simulink model "Lv_topo4"  (R2024a)
settings: Solver=ode4  StartTime=0.0  StopTime=1  FixedStep=5e-05  RelTol=1e-3
libraries: spsSeriesRLCBranchLib x38, spsThreePhaseSeriesRLCBranchLib x18, spsCurrentMeasurementLib x16, spsPowerLib x16, spsSeriesRLCLoadLib x16, spsVoltageMeasurementLib x16, spsThreePhaseVIMeasurementLib x2, spsGroundLib x2, spsPower3phInstantaneousLib x2, spsThreePhaseTransformerTwoWindingsLib x2, spsThreePhaseSourceLib x1, sps_lib x1
(part 1 of 2)
settings Model: SimulationMode=accelerator  Creator=zyx53  LastModifiedBy=zyx53
settings DataIOCC: SaveFinalState=on  SaveOperatingPoint=on  SaveState=on  ReturnWorkspaceOutputs=off

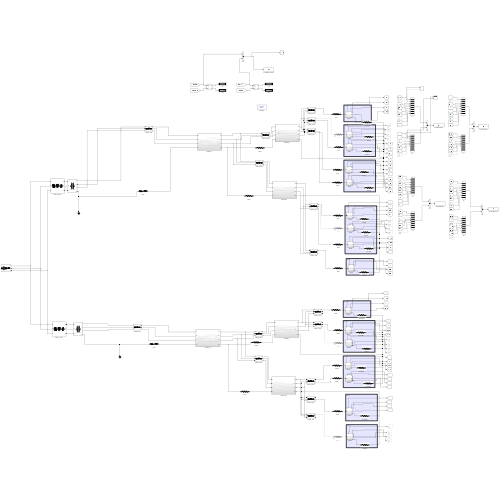
[thumbnail: Simulink's stored preview of the top-level diagram]
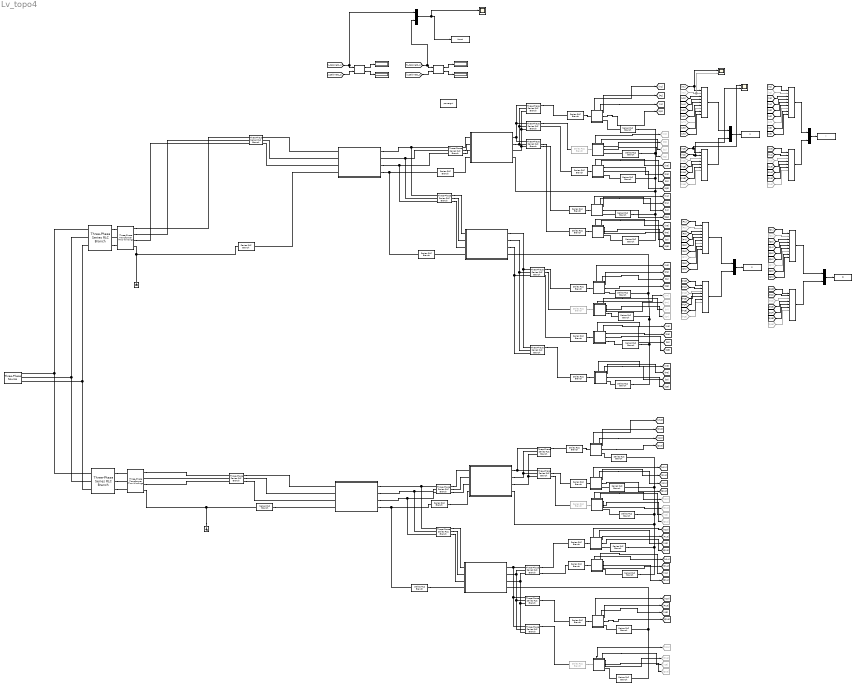
== system Lv_topo4 ==
  note: 表箱1
  note: 表箱2
  note: 表箱3
  note: 表箱4
  note: 表箱5
  note: 表箱1
  note: 表箱2
  note: 表箱3
  note: 表箱4
  note: 表箱5
  10+10m{1..2,21..22} (4 alike) : spsSeriesRLCBranchLib/Series RLC Branch  LConnTagsString=__new0  RConnTagsString=__new0  BranchType=R  Resistance=20*3.08e-3  Inductance=0  SetiL0=off  InitialCurrent=0  Capacitance=1e-6  Setx0=off  InitialVoltage=0  Measurements=None
  10+15m21 : spsSeriesRLCBranchLib/Series RLC Branch  LConnTagsString=__new0  RConnTagsString=__new0  BranchType=R  Resistance=25*3.08e-3  Inductance=0  SetiL0=off  InitialCurrent=0  Capacitance=1e-6  Setx0=off  InitialVoltage=0  Measurements=None
  10+15m24 : spsSeriesRLCBranchLib/Series RLC Branch  LConnTagsString=__new0  RConnTagsString=__new0  BranchType=R  Resistance=25*3.08e-3  Inductance=0  SetiL0=off  InitialCurrent=0  Capacitance=1e-6  Setx0=off  InitialVoltage=0  Measurements=None
  10+15m3 : spsSeriesRLCBranchLib/Series RLC Branch  LConnTagsString=__new0  RConnTagsString=__new0  BranchType=R  Resistance=25*3.08e-3  Inductance=0  SetiL0=off  InitialCurrent=0  Capacitance=1e-6  Setx0=off  InitialVoltage=0  Measurements=None
  10+5m{1..3,5,7,23} (6 alike) : spsSeriesRLCBranchLib/Series RLC Branch  LConnTagsString=__new0  RConnTagsString=__new0  BranchType=R  Resistance=15*3.08e-3  Inductance=0  SetiL0=off  InitialCurrent=0  Capacitance=1e-6  Setx0=off  InitialVoltage=0  Measurements=None
  10+7m2 : spsSeriesRLCBranchLib/Series RLC Branch  LConnTagsString=__new0  RConnTagsString=__new0  BranchType=R  Resistance=17*3.08e-3  Inductance=0  SetiL0=off  InitialCurrent=0  Capacitance=1e-6  Setx0=off  InitialVoltage=0  Measurements=None
  10m : spsSeriesRLCBranchLib/Series RLC Branch  LConnTagsString=__new0  RConnTagsString=__new0  BranchType=R  Resistance=10*3.08e-3  Inductance=0  SetiL0=off  InitialCurrent=0  Capacitance=1e-6  Setx0=off  InitialVoltage=0  Measurements=None
  10m1 : spsSeriesRLCBranchLib/Series RLC Branch  LConnTagsString=__new0  RConnTagsString=__new0  BranchType=R  Resistance=10*3.08e-3  Inductance=0  SetiL0=off  InitialCurrent=0  Capacitance=1e-6  Setx0=off  InitialVoltage=0  Measurements=None
  10m2 : spsSeriesRLCBranchLib/Series RLC Branch  LConnTagsString=__new0  RConnTagsString=__new0  BranchType=R  Resistance=10*3.08e-3  Inductance=0  SetiL0=off  InitialCurrent=0  Capacitance=1e-6  Setx0=off  InitialVoltage=0  Measurements=None
  10m21 : spsSeriesRLCBranchLib/Series RLC Branch  LConnTagsString=__new0  RConnTagsString=__new0  BranchType=R  Resistance=10*3.08e-3  Inductance=1.4e-5  SetiL0=off  InitialCurrent=0  Capacitance=1e-6  Setx0=off  InitialVoltage=0  Measurements=None
  10m22 : spsSeriesRLCBranchLib/Series RLC Branch  LConnTagsString=__new0  RConnTagsString=__new0  BranchType=R  Resistance=10*3.08e-3  Inductance=1.04e-5  SetiL0=off  InitialCurrent=0  Capacitance=1e-6  Setx0=off  InitialVoltage=0  Measurements=None
  10m24 : spsSeriesRLCBranchLib/Series RLC Branch  LConnTagsString=__new0  RConnTagsString=__new0  BranchType=R  Resistance=10*3.08e-3  Inductance=7.6e-6  SetiL0=off  InitialCurrent=0  Capacitance=1e-6  Setx0=off  InitialVoltage=0  Measurements=None
  10m26 : spsSeriesRLCBranchLib/Series RLC Branch  Commented=on  LConnTagsString=__new0  RConnTagsString=__new0  BranchType=R  Resistance=10*3.08e-3  Inductance=9.6e-6  SetiL0=off  InitialCurrent=0  Capacitance=1e-6  Setx0=off  InitialVoltage=0  Measurements=None
  10m27 : spsSeriesRLCBranchLib/Series RLC Branch  LConnTagsString=__new0  RConnTagsString=__new0  BranchType=R  Resistance=10*3.08e-3  Inductance=1.2e-5  SetiL0=off  InitialCurrent=0  Capacitance=1e-6  Setx0=off  InitialVoltage=0  Measurements=None
  10m5 : spsSeriesRLCBranchLib/Series RLC Branch  LConnTagsString=__new0  RConnTagsString=__new0  BranchType=R  Resistance=10*3.08e-3  Inductance=8.8e-6  SetiL0=off  InitialCurrent=0  Capacitance=1e-6  Setx0=off  InitialVoltage=0  Measurements=None
  10m7 : spsSeriesRLCBranchLib/Series RLC Branch  LConnTagsString=__new0  RConnTagsString=__new0  BranchType=R  Resistance=10*3.08e-3  Inductance=6e-6  SetiL0=off  InitialCurrent=0  Capacitance=1e-6  Setx0=off  InitialVoltage=0  Measurements=None
  20m1 : spsSeriesRLCBranchLib/Series RLC Branch  LConnTagsString=__new0  RConnTagsString=__new0  BranchType=R  Resistance=10*3.08e-3  Inductance=0  SetiL0=off  InitialCurrent=0  Capacitance=1e-6  Setx0=off  InitialVoltage=0  Measurements=None
  20m3 : spsSeriesRLCBranchLib/Series RLC Branch  LConnTagsString=__new0  RConnTagsString=__new0  BranchType=R  Resistance=20*3.08e-3  Inductance=0  SetiL0=off  InitialCurrent=0  Capacitance=1e-6  Setx0=off  InitialVoltage=0  Measurements=None
  25m21 : spsSeriesRLCBranchLib/Series RLC Branch  LConnTagsString=__new0  RConnTagsString=__new0  BranchType=R  Resistance=25*3.08e-3  Inductance=0  SetiL0=off  InitialCurrent=0  Capacitance=1e-6  Setx0=off  InitialVoltage=0  Measurements=None
  30m2 : spsSeriesRLCBranchLib/Series RLC Branch  LConnTagsString=__new0  RConnTagsString=__new0  BranchType=R  Resistance=30*3.08e-3  Inductance=0  SetiL0=off  InitialCurrent=0  Capacitance=1e-6  Setx0=off  InitialVoltage=0  Measurements=None
  3m2 : spsSeriesRLCBranchLib/Series RLC Branch  LConnTagsString=__new0  RConnTagsString=__new0  BranchType=RL  Resistance=0.00549  Inductance=1.2e-5  SetiL0=off  InitialCurrent=0  Capacitance=1e-6  Setx0=off  InitialVoltage=0  Measurements=None
  3m5 : spsSeriesRLCBranchLib/Series RLC Branch  LConnTagsString=__new0  RConnTagsString=__new0  BranchType=RL  Resistance=0.00549  Inductance=1.2e-5  SetiL0=off  InitialCurrent=0  Capacitance=1e-6  Setx0=off  InitialVoltage=0  Measurements=None
  5+15m25 : spsSeriesRLCBranchLib/Series RLC Branch  LConnTagsString=__new0  RConnTagsString=__new0  BranchType=R  Resistance=20*3.08e-3  Inductance=0  SetiL0=off  InitialCurrent=0  Capacitance=1e-6  Setx0=off  InitialVoltage=0  Measurements=None
  5+5m1 : spsSeriesRLCBranchLib/Series RLC Branch  LConnTagsString=__new0  RConnTagsString=__new0  BranchType=R  Resistance=10*3.08e-3  Inductance=0  SetiL0=off  InitialCurrent=0  Capacitance=1e-6  Setx0=off  InitialVoltage=0  Measurements=None
  5m : spsSeriesRLCBranchLib/Series RLC Branch  Commented=on  LConnTagsString=__new0  RConnTagsString=__new0  BranchType=R  Resistance=5*3.08e-3  Inductance=0  SetiL0=off  InitialCurrent=0  Capacitance=1e-6  Setx0=off  InitialVoltage=0  Measurements=None
  5m2 : spsSeriesRLCBranchLib/Series RLC Branch  LConnTagsString=__new0  RConnTagsString=__new0  BranchType=R  Resistance=5*3.08e-3  Inductance=0  SetiL0=off  InitialCurrent=0  Capacitance=1e-6  Setx0=off  InitialVoltage=0  Measurements=None
  5m23 : spsSeriesRLCBranchLib/Series RLC Branch  Commented=on  LConnTagsString=__new0  RConnTagsString=__new0  BranchType=R  Resistance=5*3.08e-3  Inductance=9.2e-6  SetiL0=off  InitialCurrent=0  Capacitance=1e-6  Setx0=off  InitialVoltage=0  Measurements=None
  5m25 : spsSeriesRLCBranchLib/Series RLC Branch  LConnTagsString=__new0  RConnTagsString=__new0  BranchType=R  Resistance=5*3.08e-3  Inductance=4.4e-6  SetiL0=off  InitialCurrent=0  Capacitance=1e-6  Setx0=off  InitialVoltage=0  Measurements=None
  5m3 : spsSeriesRLCBranchLib/Series RLC Branch  LConnTagsString=__new0  RConnTagsString=__new0  BranchType=R  Resistance=5*3.08e-3  Inductance=0  SetiL0=off  InitialCurrent=0  Capacitance=1e-6  Setx0=off  InitialVoltage=0  Measurements=None
  7m1 : spsSeriesRLCBranchLib/Series RLC Branch  Commented=on  LConnTagsString=__new0  RConnTagsString=__new0  BranchType=R  Resistance=7*3.08e-3  Inductance=1.2e-5  SetiL0=off  InitialCurrent=0  Capacitance=1e-6  Setx0=off  InitialVoltage=0  Measurements=None
  Cabinet1_1 : Subsystem
  Cabinet1_2 : Subsystem
  Cabinet2_1 : Subsystem
  Cabinet2_2 : Subsystem
  Cabinet2_3 : Subsystem
  Cabinet2_4 : Subsystem
  Cable1_10m1 : spsThreePhaseSeriesRLCBranchLib/Three-Phase Series RLC Branch  LConnTagsString=A|B|C  RConnTagsString=A|B|C  BranchType=RLC  Resistance=10*1.1e-7  Inductance=10*3.9e-8  Capacitance=0  Measurements=None
  Cable1_10m3 : spsThreePhaseSeriesRLCBranchLib/Three-Phase Series RLC Branch  LConnTagsString=A|B|C  RConnTagsString=A|B|C  BranchType=RLC  Resistance=10*1.1e-7  Inductance=10*3.9e-8  Capacitance=0  Measurements=None
  Cable1_10m5 : spsThreePhaseSeriesRLCBranchLib/Three-Phase Series RLC Branch  LConnTagsString=A|B|C  RConnTagsString=A|B|C  BranchType=RLC  Resistance=10*1.1e-7  Inductance=10*3.9e-8  Capacitance=0  Measurements=None
  Cable1_10m6 : spsThreePhaseSeriesRLCBranchLib/Three-Phase Series RLC Branch  LConnTagsString=A|B|C  RConnTagsString=A|B|C  BranchType=RLC  Resistance=15*1.1e-7  Inductance=15*3.9e-8  Capacitance=0  Measurements=None
  Cable1_15m1 : spsThreePhaseSeriesRLCBranchLib/Three-Phase Series RLC Branch  LConnTagsString=A|B|C  RConnTagsString=A|B|C  BranchType=RLC  Resistance=15*1.1e-7  Inductance=15*3.9e-8  Capacitance=0  Measurements=None
  Cable1_15m2 : spsThreePhaseSeriesRLCBranchLib/Three-Phase Series RLC Branch  LConnTagsString=A|B|C  RConnTagsString=A|B|C  BranchType=RLC  Resistance=15*1.1e-7  Inductance=15*3.9e-8  Capacitance=0  Measurements=None
  Cable1_15m3 : spsThreePhaseSeriesRLCBranchLib/Three-Phase Series RLC Branch  LConnTagsString=A|B|C  RConnTagsString=A|B|C  BranchType=RLC  Resistance=1.31e-3  Inductance=1.07e-3  Capacitance=0  Measurements=None
  Cable1_15m4 : spsThreePhaseSeriesRLCBranchLib/Three-Phase Series RLC Branch  LConnTagsString=A|B|C  RConnTagsString=A|B|C  BranchType=RLC  Resistance=1.31e-3  Inductance=1.07e-3  Capacitance=0  Measurements=None
  Cable1_15m5 : spsThreePhaseSeriesRLCBranchLib/Three-Phase Series RLC Branch  LConnTagsString=A|B|C  RConnTagsString=A|B|C  BranchType=RLC  Resistance=15*1.1e-7  Inductance=15*3.9e-8  Capacitance=0  Measurements=None
  Cable1_25m1 : spsThreePhaseSeriesRLCBranchLib/Three-Phase Series RLC Branch  LConnTagsString=A|B|C  RConnTagsString=A|B|C  BranchType=RLC  Resistance=25*1.1e-7  Inductance=25*3.9e-8  Capacitance=0  Measurements=None
  Cable1_30m2 : spsThreePhaseSeriesRLCBranchLib/Three-Phase Series RLC Branch  LConnTagsString=A|B|C  RConnTagsString=A|B|C  BranchType=RLC  Resistance=30*1.1e-7  Inductance=30*3.9e-8  Capacitance=0  Measurements=None
  Cable1_3m2 : spsThreePhaseSeriesRLCBranchLib/Three-Phase Series RLC Branch  LConnTagsString=A|B|C  RConnTagsString=A|B|C  BranchType=RLC  Resistance=0.000804  Inductance=0  Capacitance=0  Measurements=None
  Cable1_5m1 : spsThreePhaseSeriesRLCBranchLib/Three-Phase Series RLC Branch  LConnTagsString=A|B|C  RConnTagsString=A|B|C  BranchType=RLC  Resistance=5*1.1e-7  Inductance=5*3.9e-8  Capacitance=0  Measurements=None
  Cable1_5m2 : spsThreePhaseSeriesRLCBranchLib/Three-Phase Series RLC Branch  LConnTagsString=A|B|C  RConnTagsString=A|B|C  BranchType=RLC  Resistance=5*1.1e-7  Inductance=5*3.9e-8  Capacitance=0  Measurements=None
  Cable1_5m7 : spsThreePhaseSeriesRLCBranchLib/Three-Phase Series RLC Branch  LConnTagsString=A|B|C  RConnTagsString=A|B|C  BranchType=RLC  Resistance=15*1.1e-7  Inductance=15*3.9e-8  Capacitance=0  Measurements=None
  Cable2_10m1 : spsThreePhaseSeriesRLCBranchLib/Three-Phase Series RLC Branch  LConnTagsString=A|B|C  RConnTagsString=A|B|C  BranchType=RLC  Resistance=10*1.1e-7  Inductance=10*3.9e-8  Capacitance=0  Measurements=None
  Cable2_20m : spsThreePhaseSeriesRLCBranchLib/Three-Phase Series RLC Branch  LConnTagsString=A|B|C  RConnTagsString=A|B|C  BranchType=RLC  Resistance=20*1.1e-7  Inductance=20*3.9e-8  Capacitance=0  Measurements=None
  Cable2_2m2 : spsThreePhaseSeriesRLCBranchLib/Three-Phase Series RLC Branch  LConnTagsString=A|B|C  RConnTagsString=A|B|C  BranchType=RLC  Resistance=0.000536  Inductance=0  Capacitance=0  Measurements=None
  From12 : From  Commented=on  GotoTag=P2
  From17 : From  Commented=on  GotoTag=P7
  From2 : From  Commented=on  GotoTag=V2
  From21 : From  Commented=on  GotoTag=I2
  From26 : From  Commented=on  GotoTag=I7
  From30 : From  Commented=on  GotoTag=Q2
  From35 : From  Commented=on  GotoTag=Q7
  From43 : From  Commented=on  GotoTag=P12
  From47 : From  Commented=on  GotoTag=P16
  From51 : From  Commented=on  GotoTag=I12
  From55 : From  Commented=on  GotoTag=I16
  From57 : From  Commented=on  GotoTag=V12
  From59 : From  Commented=on  GotoTag=Q12
  From63 : From  Commented=on  GotoTag=Q16
  From67 : From  Commented=on  GotoTag=V16
  From7 : From  Commented=on  GotoTag=V7
  Goto1 : Goto  Commented=on  GotoTag=V2
  Goto10 : Goto  Commented=on  GotoTag=P2
  Goto15 : Goto  Commented=on  GotoTag=P7
  Goto19 : Goto  Commented=on  GotoTag=I2
  Goto24 : Goto  Commented=on  GotoTag=I7
  Goto28 : Goto  Commented=on  GotoTag=Q2
  Goto33 : Goto  Commented=on  GotoTag=Q7
  Goto39 : Goto  Commented=on  GotoTag=P12
  Goto43 : Goto  Commented=on  GotoTag=P16
  Goto46 : Goto  Commented=on  GotoTag=V12
  Goto47 : Goto  Commented=on  GotoTag=I12
  Goto51 : Goto  Commented=on  GotoTag=I16
  Goto54 : Goto  Commented=on  GotoTag=Q12
  Goto59 : Goto  Commented=on  GotoTag=Q16
  Goto6 : Goto  Commented=on  GotoTag=V7
  Goto62 : Goto  Commented=on  GotoTag=V16
  Ground : spsGroundLib/Ground  LConnTagsString=a
  Ground1 : spsGroundLib/Ground  LConnTagsString=a
  I : Concatenate  NumInputs=9
  I1 : Concatenate  NumInputs=9
  P : Concatenate  NumInputs=9
  P1 : Concatenate  NumInputs=9
  P2 : Display
  P9 : Display
  "Power (3ph, Instantaneous)" : spsPower3phInstantaneousLib/Power (3ph, Instantaneous)
  "Power (3ph, Instantaneous)1" : spsPower3phInstantaneousLib/Power (3ph, Instantaneous)
  Q : Concatenate  NumInputs=9
  Q1 : Concatenate  NumInputs=9
  Q2 : Display
  Q9 : Display
  Scope : Scope  NumInputPorts=2
  Scope1 : Scope  NumInputPorts=2
  Scope2 : Scope
  Three-Phase Transformer (Two Windings) : spsThreePhaseTransformerTwoWindingsLib/Three-Phase Transformer (Two Windings)  Winding1Connection=Yg  Winding2Connection=Yn  CoreType=Three single-phase transformers  SetSaturation=off  Hysteresis=off  DataFile='hysteresis'  SetInitialFlux=off  Measurements=None  UNITS=SI  NominalPower=[ 100000 , 50 ]  Winding1=[10000 , 0 , 0]  Winding2=[400 , 0.084 , 8.05e-4]  Rm=1500  Lm=1.2  L0=0.5  Saturation=[0 0;0.66653 1910.3;277.72 2419.7]  InitialFluxes=[ 0.8 , -0.8 , 0.7 ]  BreakLoop=off  DiscreteSolver=Trapezoidal iterative  DataType=on  TransfoNumber=1
  Three-Phase Transformer (Two Windings)2 : spsThreePhaseTransformerTwoWindingsLib/Three-Phase Transformer (Two Windings)  Winding1Connection=Yg  Winding2Connection=Yn  CoreType=Three single-phase transformers  SetSaturation=off  Hysteresis=off  DataFile='hysteresis'  SetInitialFlux=off  Measurements=None  UNITS=SI  NominalPower=[ 100000 , 50 ]  Winding1=[10000 , 0 , 0]  Winding2=[400 , 0.084 , 8.05e-4]  Rm=1500  Lm=1.2  L0=0.5  Saturation=[0 0;0.66653 1910.3;277.72 2419.7]  InitialFluxes=[ 0.8 , -0.8 , 0.7 ]  BreakLoop=off  DiscreteSolver=Trapezoidal iterative  DataType=on  TransfoNumber=1
  Three-Phase Source : spsThreePhaseSourceLib/Three-Phase Source  InternalConnection=Yg  VoltagePhases=off  Voltage=10e3  PhaseAngle=0  Voltage_phases=[25e3 25e3 25e3]/sqrt(3)  PhaseAngles_phases=[0 -120 +120]  Frequency=50  NonIdealSource=on  SpecifyImpedance=off  Resistance=0.01  Inductance=0.001  ShortCircuitLevel=30e6  BaseVoltage=10e3  XRratio=7  BusType=swing  Pref=10e3  Qref=0  Prefabc=[10e3, 10e3, 10e3]  Qrefabc=[0, 0, 0]  Qmin=-inf  Qmax=inf
  To Workspace I : ToWorkspace  VariableName=I  SaveFormat=Timeseries  SampleTime=-1
  To Workspace P : ToWorkspace  VariableName=P  SaveFormat=Timeseries  SampleTime=-1
  To Workspace Q : ToWorkspace  VariableName=Q  SaveFormat=Timeseries  SampleTime=-1
  To Workspace U : ToWorkspace  VariableName=U  SaveFormat=Timeseries  SampleTime=-1
  To Workspace Uroot : ToWorkspace  VariableName=Uroot  SaveFormat=Timeseries  SampleTime=-1
  U : Concatenate  NumInputs=9
  U1 : Concatenate  NumInputs=9
  U{2..6} (5 alike) : Concatenate
  User1 : Subsystem
      settings: PortSchema="{\"entries\":[{\"content\":{\"sides\":[{\"content\":{\"connectorIds\":[\"LConn1\"]},\"type\":\"ConnectorPlacement.EquallySpacedRectSide\",\"uuid\":\"108acfb9-5be9-46f7-bd10-3aae17a40b63\"},{\"content\":{\"connectorIds\":[\"Out1\",\"Out2\",\"RConn1\"],\"side\":\"RIGHT\"},\"type\":\"ConnectorPlacement.EquallySpacedRectSide\",\"uuid\":\"d21e5312-b16e-4825-8d19-93c29509c0ff\"},{\"content\":{\"connectorIds\":[\"Out3\",\"Out4\"],\"side\":\"TOP\"},\"type\":\"ConnectorPlacement.EquallySpacedRectSide\",\"uuid\":\"46703d4a-0476-4df2-9aa7-7e20b378624b\"}]},\"type\":\"ConnectorPlacement.EquallySpacedConnector\",\"uuid\":\"ca4322da-2652-4337-be60-49b74a2e02a6\"}],\"packageUris\":[\"http://schema.mathworks.com/mf0/Connector/R2020b\"],\"version\":\"1.0\"}"
  User10 : Subsystem
      settings: PortSchema="{\"entries\":[{\"content\":{\"sides\":[{\"content\":{\"connectorIds\":[\"LConn1\"]},\"type\":\"ConnectorPlacement.EquallySpacedRectSide\",\"uuid\":\"108acfb9-5be9-46f7-bd10-3aae17a40b63\"},{\"content\":{\"connectorIds\":[\"Out1\",\"Out2\",\"RConn1\"],\"side\":\"RIGHT\"},\"type\":\"ConnectorPlacement.EquallySpacedRectSide\",\"uuid\":\"d21e5312-b16e-4825-8d19-93c29509c0ff\"},{\"content\":{\"connectorIds\":[\"Out3\",\"Out4\"],\"side\":\"TOP\"},\"type\":\"ConnectorPlacement.EquallySpacedRectSide\",\"uuid\":\"46703d4a-0476-4df2-9aa7-7e20b378624b\"}]},\"type\":\"ConnectorPlacement.EquallySpacedConnector\",\"uuid\":\"ca4322da-2652-4337-be60-49b74a2e02a6\"}],\"packageUris\":[\"http://schema.mathworks.com/mf0/Connector/R2020b\"],\"version\":\"1.0\"}"
  User11 : Subsystem
      settings: PortSchema="{\"entries\":[{\"content\":{\"sides\":[{\"content\":{\"connectorIds\":[\"LConn1\"]},\"type\":\"ConnectorPlacement.EquallySpacedRectSide\",\"uuid\":\"108acfb9-5be9-46f7-bd10-3aae17a40b63\"},{\"content\":{\"connectorIds\":[\"Out1\",\"Out2\",\"RConn1\"],\"side\":\"RIGHT\"},\"type\":\"ConnectorPlacement.EquallySpacedRectSide\",\"uuid\":\"d21e5312-b16e-4825-8d19-93c29509c0ff\"},{\"content\":{\"connectorIds\":[\"Out3\",\"Out4\"],\"side\":\"TOP\"},\"type\":\"ConnectorPlacement.EquallySpacedRectSide\",\"uuid\":\"46703d4a-0476-4df2-9aa7-7e20b378624b\"}]},\"type\":\"ConnectorPlacement.EquallySpacedConnector\",\"uuid\":\"ca4322da-2652-4337-be60-49b74a2e02a6\"}],\"packageUris\":[\"http://schema.mathworks.com/mf0/Connector/R2020b\"],\"version\":\"1.0\"}"
  User12 : Subsystem
      settings: PortSchema="{\"entries\":[{\"content\":{\"sides\":[{\"content\":{\"connectorIds\":[\"LConn1\"]},\"type\":\"ConnectorPlacement.EquallySpacedRectSide\",\"uuid\":\"108acfb9-5be9-46f7-bd10-3aae17a40b63\"},{\"content\":{\"connectorIds\":[\"Out1\",\"Out2\",\"RConn1\"],\"side\":\"RIGHT\"},\"type\":\"ConnectorPlacement.EquallySpacedRectSide\",\"uuid\":\"d21e5312-b16e-4825-8d19-93c29509c0ff\"},{\"content\":{\"connectorIds\":[\"Out3\",\"Out4\"],\"side\":\"TOP\"},\"type\":\"ConnectorPlacement.EquallySpacedRectSide\",\"uuid\":\"46703d4a-0476-4df2-9aa7-7e20b378624b\"}]},\"type\":\"ConnectorPlacement.EquallySpacedConnector\",\"uuid\":\"ca4322da-2652-4337-be60-49b74a2e02a6\"}],\"packageUris\":[\"http://schema.mathworks.com/mf0/Connector/R2020b\"],\"version\":\"1.0\"}"
  User13 : Subsystem
      settings: PortSchema="{\"entries\":[{\"content\":{\"sides\":[{\"content\":{\"connectorIds\":[\"LConn1\"]},\"type\":\"ConnectorPlacement.EquallySpacedRectSide\",\"uuid\":\"108acfb9-5be9-46f7-bd10-3aae17a40b63\"},{\"content\":{\"connectorIds\":[\"Out1\",\"Out2\",\"RConn1\"],\"side\":\"RIGHT\"},\"type\":\"ConnectorPlacement.EquallySpacedRectSide\",\"uuid\":\"d21e5312-b16e-4825-8d19-93c29509c0ff\"},{\"content\":{\"connectorIds\":[\"Out3\",\"Out4\"],\"side\":\"TOP\"},\"type\":\"ConnectorPlacement.EquallySpacedRectSide\",\"uuid\":\"46703d4a-0476-4df2-9aa7-7e20b378624b\"}]},\"type\":\"ConnectorPlacement.EquallySpacedConnector\",\"uuid\":\"ca4322da-2652-4337-be60-49b74a2e02a6\"}],\"packageUris\":[\"http://schema.mathworks.com/mf0/Connector/R2020b\"],\"version\":\"1.0\"}"
  User14 : Subsystem
      settings: PortSchema="{\"entries\":[{\"content\":{\"sides\":[{\"content\":{\"connectorIds\":[\"LConn1\"]},\"type\":\"ConnectorPlacement.EquallySpacedRectSide\",\"uuid\":\"108acfb9-5be9-46f7-bd10-3aae17a40b63\"},{\"content\":{\"connectorIds\":[\"Out1\",\"Out2\",\"RConn1\"],\"side\":\"RIGHT\"},\"type\":\"ConnectorPlacement.EquallySpacedRectSide\",\"uuid\":\"d21e5312-b16e-4825-8d19-93c29509c0ff\"},{\"content\":{\"connectorIds\":[\"Out3\",\"Out4\"],\"side\":\"TOP\"},\"type\":\"ConnectorPlacement.EquallySpacedRectSide\",\"uuid\":\"46703d4a-0476-4df2-9aa7-7e20b378624b\"}]},\"type\":\"ConnectorPlacement.EquallySpacedConnector\",\"uuid\":\"ca4322da-2652-4337-be60-49b74a2e02a6\"}],\"packageUris\":[\"http://schema.mathworks.com/mf0/Connector/R2020b\"],\"version\":\"1.0\"}"
  User15 : Subsystem
      settings: PortSchema="{\"entries\":[{\"content\":{\"sides\":[{\"content\":{\"connectorIds\":[\"LConn1\"]},\"type\":\"ConnectorPlacement.EquallySpacedRectSide\",\"uuid\":\"108acfb9-5be9-46f7-bd10-3aae17a40b63\"},{\"content\":{\"connectorIds\":[\"Out1\",\"Out2\",\"RConn1\"],\"side\":\"RIGHT\"},\"type\":\"ConnectorPlacement.EquallySpacedRectSide\",\"uuid\":\"d21e5312-b16e-4825-8d19-93c29509c0ff\"},{\"content\":{\"connectorIds\":[\"Out3\",\"Out4\"],\"side\":\"TOP\"},\"type\":\"ConnectorPlacement.EquallySpacedRectSide\",\"uuid\":\"46703d4a-0476-4df2-9aa7-7e20b378624b\"}]},\"type\":\"ConnectorPlacement.EquallySpacedConnector\",\"uuid\":\"ca4322da-2652-4337-be60-49b74a2e02a6\"}],\"packageUris\":[\"http://schema.mathworks.com/mf0/Connector/R2020b\"],\"version\":\"1.0\"}"
  User16 : Subsystem
      settings: PortSchema="{\"entries\":[{\"content\":{\"sides\":[{\"content\":{\"connectorIds\":[\"LConn1\"]},\"type\":\"ConnectorPlacement.EquallySpacedRectSide\",\"uuid\":\"108acfb9-5be9-46f7-bd10-3aae17a40b63\"},{\"content\":{\"connectorIds\":[\"Out1\",\"Out2\",\"RConn1\"],\"side\":\"RIGHT\"},\"type\":\"ConnectorPlacement.EquallySpacedRectSide\",\"uuid\":\"d21e5312-b16e-4825-8d19-93c29509c0ff\"},{\"content\":{\"connectorIds\":[\"Out3\",\"Out4\"],\"side\":\"TOP\"},\"type\":\"ConnectorPlacement.EquallySpacedRectSide\",\"uuid\":\"46703d4a-0476-4df2-9aa7-7e20b378624b\"}]},\"type\":\"ConnectorPlacement.EquallySpacedConnector\",\"uuid\":\"ca4322da-2652-4337-be60-49b74a2e02a6\"}],\"packageUris\":[\"http://schema.mathworks.com/mf0/Connector/R2020b\"],\"version\":\"1.0\"}"
  User2 : Subsystem
      settings: PortSchema="{\"entries\":[{\"content\":{\"sides\":[{\"content\":{\"connectorIds\":[\"LConn1\"]},\"type\":\"ConnectorPlacement.EquallySpacedRectSide\",\"uuid\":\"108acfb9-5be9-46f7-bd10-3aae17a40b63\"},{\"content\":{\"connectorIds\":[\"Out1\",\"Out2\",\"RConn1\"],\"side\":\"RIGHT\"},\"type\":\"ConnectorPlacement.EquallySpacedRectSide\",\"uuid\":\"d21e5312-b16e-4825-8d19-93c29509c0ff\"},{\"content\":{\"connectorIds\":[\"Out3\",\"Out4\"],\"side\":\"TOP\"},\"type\":\"ConnectorPlacement.EquallySpacedRectSide\",\"uuid\":\"46703d4a-0476-4df2-9aa7-7e20b378624b\"}]},\"type\":\"ConnectorPlacement.EquallySpacedConnector\",\"uuid\":\"ca4322da-2652-4337-be60-49b74a2e02a6\"}],\"packageUris\":[\"http://schema.mathworks.com/mf0/Connector/R2020b\"],\"version\":\"1.0\"}"
  User3 : Subsystem
      settings: PortSchema="{\"entries\":[{\"content\":{\"sides\":[{\"content\":{\"connectorIds\":[\"LConn1\"]},\"type\":\"ConnectorPlacement.EquallySpacedRectSide\",\"uuid\":\"108acfb9-5be9-46f7-bd10-3aae17a40b63\"},{\"content\":{\"connectorIds\":[\"Out1\",\"Out2\",\"RConn1\"],\"side\":\"RIGHT\"},\"type\":\"ConnectorPlacement.EquallySpacedRectSide\",\"uuid\":\"d21e5312-b16e-4825-8d19-93c29509c0ff\"},{\"content\":{\"connectorIds\":[\"Out3\",\"Out4\"],\"side\":\"TOP\"},\"type\":\"ConnectorPlacement.EquallySpacedRectSide\",\"uuid\":\"46703d4a-0476-4df2-9aa7-7e20b378624b\"}]},\"type\":\"ConnectorPlacement.EquallySpacedConnector\",\"uuid\":\"ca4322da-2652-4337-be60-49b74a2e02a6\"}],\"packageUris\":[\"http://schema.mathworks.com/mf0/Connector/R2020b\"],\"version\":\"1.0\"}"
  User4 : Subsystem
      settings: PortSchema="{\"entries\":[{\"content\":{\"sides\":[{\"content\":{\"connectorIds\":[\"LConn1\"]},\"type\":\"ConnectorPlacement.EquallySpacedRectSide\",\"uuid\":\"108acfb9-5be9-46f7-bd10-3aae17a40b63\"},{\"content\":{\"connectorIds\":[\"Out1\",\"Out2\",\"RConn1\"],\"side\":\"RIGHT\"},\"type\":\"ConnectorPlacement.EquallySpacedRectSide\",\"uuid\":\"d21e5312-b16e-4825-8d19-93c29509c0ff\"},{\"content\":{\"connectorIds\":[\"Out3\",\"Out4\"],\"side\":\"TOP\"},\"type\":\"ConnectorPlacement.EquallySpacedRectSide\",\"uuid\":\"46703d4a-0476-4df2-9aa7-7e20b378624b\"}]},\"type\":\"ConnectorPlacement.EquallySpacedConnector\",\"uuid\":\"ca4322da-2652-4337-be60-49b74a2e02a6\"}],\"packageUris\":[\"http://schema.mathworks.com/mf0/Connector/R2020b\"],\"version\":\"1.0\"}"
  User5 : Subsystem
      settings: PortSchema="{\"entries\":[{\"content\":{\"sides\":[{\"content\":{\"connectorIds\":[\"LConn1\"]},\"type\":\"ConnectorPlacement.EquallySpacedRectSide\",\"uuid\":\"108acfb9-5be9-46f7-bd10-3aae17a40b63\"},{\"content\":{\"connectorIds\":[\"Out1\",\"Out2\",\"RConn1\"],\"side\":\"RIGHT\"},\"type\":\"ConnectorPlacement.EquallySpacedRectSide\",\"uuid\":\"d21e5312-b16e-4825-8d19-93c29509c0ff\"},{\"content\":{\"connectorIds\":[\"Out3\",\"Out4\"],\"side\":\"TOP\"},\"type\":\"ConnectorPlacement.EquallySpacedRectSide\",\"uuid\":\"46703d4a-0476-4df2-9aa7-7e20b378624b\"}]},\"type\":\"ConnectorPlacement.EquallySpacedConnector\",\"uuid\":\"ca4322da-2652-4337-be60-49b74a2e02a6\"}],\"packageUris\":[\"http://schema.mathworks.com/mf0/Connector/R2020b\"],\"version\":\"1.0\"}"
  User6 : Subsystem
      settings: PortSchema="{\"entries\":[{\"content\":{\"sides\":[{\"content\":{\"connectorIds\":[\"LConn1\"]},\"type\":\"ConnectorPlacement.EquallySpacedRectSide\",\"uuid\":\"108acfb9-5be9-46f7-bd10-3aae17a40b63\"},{\"content\":{\"connectorIds\":[\"Out1\",\"Out2\",\"RConn1\"],\"side\":\"RIGHT\"},\"type\":\"ConnectorPlacement.EquallySpacedRectSide\",\"uuid\":\"d21e5312-b16e-4825-8d19-93c29509c0ff\"},{\"content\":{\"connectorIds\":[\"Out3\",\"Out4\"],\"side\":\"TOP\"},\"type\":\"ConnectorPlacement.EquallySpacedRectSide\",\"uuid\":\"46703d4a-0476-4df2-9aa7-7e20b378624b\"}]},\"type\":\"ConnectorPlacement.EquallySpacedConnector\",\"uuid\":\"ca4322da-2652-4337-be60-49b74a2e02a6\"}],\"packageUris\":[\"http://schema.mathworks.com/mf0/Connector/R2020b\"],\"version\":\"1.0\"}"
  User7 : Subsystem
      settings: PortSchema="{\"entries\":[{\"content\":{\"sides\":[{\"content\":{\"connectorIds\":[\"LConn1\"]},\"type\":\"ConnectorPlacement.EquallySpacedRectSide\",\"uuid\":\"108acfb9-5be9-46f7-bd10-3aae17a40b63\"},{\"content\":{\"connectorIds\":[\"Out1\",\"Out2\",\"RConn1\"],\"side\":\"RIGHT\"},\"type\":\"ConnectorPlacement.EquallySpacedRectSide\",\"uuid\":\"d21e5312-b16e-4825-8d19-93c29509c0ff\"},{\"content\":{\"connectorIds\":[\"Out3\",\"Out4\"],\"side\":\"TOP\"},\"type\":\"ConnectorPlacement.EquallySpacedRectSide\",\"uuid\":\"46703d4a-0476-4df2-9aa7-7e20b378624b\"}]},\"type\":\"ConnectorPlacement.EquallySpacedConnector\",\"uuid\":\"ca4322da-2652-4337-be60-49b74a2e02a6\"}],\"packageUris\":[\"http://schema.mathworks.com/mf0/Connector/R2020b\"],\"version\":\"1.0\"}"
  User8 : Subsystem
      settings: PortSchema="{\"entries\":[{\"content\":{\"sides\":[{\"content\":{\"connectorIds\":[\"LConn1\"]},\"type\":\"ConnectorPlacement.EquallySpacedRectSide\",\"uuid\":\"108acfb9-5be9-46f7-bd10-3aae17a40b63\"},{\"content\":{\"connectorIds\":[\"Out1\",\"Out2\",\"RConn1\"],\"side\":\"RIGHT\"},\"type\":\"ConnectorPlacement.EquallySpacedRectSide\",\"uuid\":\"d21e5312-b16e-4825-8d19-93c29509c0ff\"},{\"content\":{\"connectorIds\":[\"Out3\",\"Out4\"],\"side\":\"TOP\"},\"type\":\"ConnectorPlacement.EquallySpacedRectSide\",\"uuid\":\"46703d4a-0476-4df2-9aa7-7e20b378624b\"}]},\"type\":\"ConnectorPlacement.EquallySpacedConnector\",\"uuid\":\"ca4322da-2652-4337-be60-49b74a2e02a6\"}],\"packageUris\":[\"http://schema.mathworks.com/mf0/Connector/R2020b\"],\"version\":\"1.0\"}"
  User9 : Subsystem
      settings: PortSchema="{\"entries\":[{\"content\":{\"sides\":[{\"content\":{\"connectorIds\":[\"LConn1\"]},\"type\":\"ConnectorPlacement.EquallySpacedRectSide\",\"uuid\":\"108acfb9-5be9-46f7-bd10-3aae17a40b63\"},{\"content\":{\"connectorIds\":[\"Out1\",\"Out2\",\"RConn1\"],\"side\":\"RIGHT\"},\"type\":\"ConnectorPlacement.EquallySpacedRectSide\",\"uuid\":\"d21e5312-b16e-4825-8d19-93c29509c0ff\"},{\"content\":{\"connectorIds\":[\"Out3\",\"Out4\"],\"side\":\"TOP\"},\"type\":\"ConnectorPlacement.EquallySpacedRectSide\",\"uuid\":\"46703d4a-0476-4df2-9aa7-7e20b378624b\"}]},\"type\":\"ConnectorPlacement.EquallySpacedConnector\",\"uuid\":\"ca4322da-2652-4337-be60-49b74a2e02a6\"}],\"packageUris\":[\"http://schema.mathworks.com/mf0/Connector/R2020b\"],\"version\":\"1.0\"}"
  powergui : sps_lib/powergui  Priority=1  SimulationMode=Discrete  SampleTime=50e-6  frequency=50  Iterations=50  frequencyindice=50  Pbase=100e6  ErrMax=1e-4  UnitsV=kV  UnitsW=MW  buscounter=2  FunctionMessages=off  echomessages=off  EnableUseOfTLC=off  CurrentSourceSwitches=off  DisableSnubberDevices=off  DisableRonSwitches=off  DisableVfSwitches=off  DisplayEquations=off  AutomaticDiscreteSolvers=off  SolverType=Tustin/Backward Euler (TBE)  Interpol=off  ExternalGateDelay=off  methode=off  Ts=100  x0status=blocks  SPID=on  SwTol=0  HookPort=off  NonlinearTolerance=1e-4  nMaxIteration=100  ContinueOnMaxIteration=off  RestoreLinks=warning  ResistiveCurrentMeasurement=off  Frange=[0:2:500]  Ylog=off  Xlog=on  ShowGrid=off  save=off  variable=ZData  structure=0  ZoomFFT=off  StartTime=0.0  cycles=1  DisplayStyle=1  fundamental=60  FreqAxis=off  MaxFrequency=1000  frequencyindicesteady=1  RmsSteady=1  display=off
  wires:
  User1/3(V) -> [V1]
  User1/4(I) -> [I1]
  User1/1(P) -> [P1]
  User1/2(Q) -> [Q1]
  User2/3(V) -> Goto1/1
  User2/4(I) -> Goto19/1
  User2/2(Q) -> Goto28/1
  User2/1(P) -> Goto10/1
  User3/4(I) -> [I3]
  User3/3(V) -> [V3]
  User3/2(Q) -> [Q3]
  User4/3(V) -> [V4]
  User4/1(P) -> [P4]
  User5/2(Q) -> [Q5]
  User5/4(I) -> [I5]
  User5/3(V) -> [V5]
  User5/1(P) -> [P5]
  User6/4(I) -> [I6]
  User6/3(V) -> [V6]
  User6/1(P) -> [P6]
  User7/2(Q) -> Goto33/1
  User7/4(I) -> Goto24/1
  User6/2(Q) -> [Q6]
  User7/3(V) -> Goto6/1
  User7/1(P) -> Goto15/1
  User8/3(V) -> [V8]
  User8/2(Q) -> [Q8]
  User8/1(P) -> [P8]
  User8/4(I) -> [I8]
  [I_Cabinet1_1] -> "Power (3ph, Instantaneous)"/2
  "Power (3ph, Instantaneous)"/1 -> P9/1
  "Power (3ph, Instantaneous)"/2 -> Q9/1
  User9/3(V) -> [V9]
  User9/1(P) -> [P9]
  User9/2(Q) -> [Q9]
  User9/4(I) -> [I9]
  [V1] -> U/1, Scope/1
  From2/1 -> Scope/2, U/2
  [V3] -> U/3
  [V4] -> U/4
  [V5] -> U/5
  [V6] -> U/6
  From7/1 -> U/7
  [V8] -> U/8
  [V9] -> U/9
  User3/1(P) -> [P3]
  User4/4(I) -> [I4]
  [P4] -> P/4
  [P3] -> P/3
  [P9] -> P/9
  From17/1 -> P/7
  [P6] -> P/6
  [P8] -> P/8
  [P1] -> P/1
  From12/1 -> P/2
  [P5] -> P/5
  [I4] -> I/4
  [I3] -> I/3
  [I9] -> I/9
  From26/1 -> I/7
  [I6] -> I/6
  [I8] -> I/8
  [I1] -> I/1
  From21/1 -> I/2
  [I5] -> I/5
  [Q4] -> Q/4
  [Q3] -> Q/3
  [Q9] -> Q/9
  From35/1 -> Q/7
  [Q6] -> Q/6
  [Q8] -> Q/8
  [Q1] -> Q/1
  From30/1 -> Q/2
  [Q5] -> Q/5
  [P11] -> P1/2
  User16/1(P) -> Goto43/1
  [I11] -> I1/2
  [Q13] -> Q1/4
  [P10] -> P1/1
  From47/1 -> P1/7
  [I14] -> I1/5
  User12/1(P) -> Goto39/1
  User14/2(Q) -> [Q14]
  From43/1 -> P1/3
  [I10] -> I1/1
  User13/4(I) -> [I13]
  From67/1 -> U1/7
  User10/1(P) -> [P10]
  U1/1 -> U2/2
  [I13] -> I1/4
  User16/3(V) -> Goto62/1
  User10/4(I) -> [I10]
  From51/1 -> I1/3
  [P13] -> P1/4
  From57/1 -> U1/3
  [V13] -> U1/4
  "Power (3ph, Instantaneous)1"/1 -> P2/1
  User11/3(V) -> [V11]
  User14/3(V) -> [V14]
  User15/2(Q) -> [Q15]
  "Power (3ph, Instantaneous)1"/2 -> Q2/1
  User16/2(Q) -> Goto59/1
  User13/1(P) -> [P13]
  User16/4(I) -> Goto51/1
  User15/4(I) -> [I15]
  User13/2(Q) -> [Q13]
  User12/2(Q) -> Goto54/1
  User13/3(V) -> [V13]
  User12/3(V) -> Goto46/1
  User12/4(I) -> Goto47/1
  User10/3(V) -> [V10]
  User15/3(V) -> [V15]
  User10/2(Q) -> [Q10]
  User14/4(I) -> [I14]
  [Q10] -> Q1/1
  [V15] -> U1/6
  [Q15] -> Q1/6
  [Q14] -> Q1/5
  [P14] -> P1/5
  User15/1(P) -> [P15]
  User14/1(P) -> [P14]
  [I_Cabinet2_1] -> "Power (3ph, Instantaneous)1"/2
  [P15] -> P1/6
  From55/1 -> I1/7
  [I15] -> I1/6
  User11/2(Q) -> [Q11]
  [V14] -> U1/5
  From59/1 -> Q1/3
  User11/1(P) -> [P11]
  [Q11] -> Q1/2
  From63/1 -> Q1/7
  I1/1 -> U3/2
  User11/4(I) -> [I11]
  U2/1 -> To Workspace U/1
  U/1 -> U2/1
  U3/1 -> To Workspace I/1
  I/1 -> U3/1
  P1/1 -> U4/2
  U4/1 -> To Workspace P/1
  P/1 -> U4/1
  Q1/1 -> U5/2
  U5/1 -> To Workspace Q/1
  Q/1 -> U5/1
  [V_Cabinet2_1] -> U6/2, "Power (3ph, Instantaneous)1"/1
  U6/1 -> Scope2/1, To Workspace Uroot/1
  [V_Cabinet1_1] -> U6/1, "Power (3ph, Instantaneous)"/1
  [V11] -> Scope1/2, U1/2
  [V10] -> Scope1/1, U1/1
  User4/2(Q) -> [Q4]
  connections:
  Cable1_15m2/RConn1 -- 10m/LConn1
  3m2/LConn1 -- Ground/LConn1 -- Three-Phase Transformer (Two Windings)/RConn4
  Cable1_30m2/RConn2 -- Cabinet2_1/LConn2
  Cable1_30m2/RConn3 -- Cabinet2_1/LConn3
  Cable1_15m2/LConn1 -- Cable1_5m1/LConn1 -- Cabinet2_1/RConn1 -- Cable1_10m3/LConn1
  Cable1_15m2/LConn2 -- Cable1_5m1/LConn2 -- Cabinet2_1/RConn2 -- Cable1_10m3/LConn2
  Cable1_15m2/LConn3 -- Cable1_10m3/LConn3 -- Cable1_5m1/LConn3 -- Cabinet2_1/RConn3
  Cabinet2_2/LConn4 -- 20m3/RConn1
  10+10m1/LConn1 -- User3/RConn1
  Cable1_10m1/LConn3 -- Cabinet2_2/RConn3 -- Cable1_5m2/LConn3
  Cable2_20m/RConn3 -- Cabinet2_2/LConn3
  Cable2_20m/RConn1 -- Cabinet2_2/LConn1
  Cable1_10m1/LConn2 -- Cabinet2_2/RConn2 -- Cable1_5m2/LConn2
  Cable2_20m/RConn2 -- Cabinet2_2/LConn2
  Cable1_10m1/LConn1 -- Cabinet2_2/RConn1 -- Cable1_5m2/LConn1
  10m5/LConn1 -- Cable1_10m1/RConn3
  User8/RConn1 -- 10+10m2/LConn1
  5m/RConn1 -- User2/LConn1
  10m1/RConn1 -- User3/LConn1
  5m2/RConn1 -- User4/LConn1
  10m2/RConn1 -- User5/LConn1
  5m3/RConn1 -- User6/LConn1
  Cable1_10m1/RConn1 -- 5m3/LConn1
  7m1/RConn1 -- User7/LConn1
  Cable1_10m1/RConn2 -- 7m1/LConn1
  10m5/RConn1 -- User8/LConn1
  10m7/RConn1 -- User9/LConn1
  10m/RConn1 -- User1/LConn1
  10+5m23/LConn1 -- User16/RConn1
  5+15m25/LConn1 -- User14/RConn1
  Cable2_10m1/LConn1 -- Cabinet1_2/RConn1 -- Cable1_25m1/LConn1
  Cabinet1_2/RConn4 -- 20m1/LConn1 -- 25m21/LConn1
  Cable2_10m1/LConn2 -- Cabinet1_2/RConn2 -- Cable1_25m1/LConn2
  Cable2_10m1/LConn3 -- Cabinet1_2/RConn3 -- Cable1_25m1/LConn3
  Cable2_10m1/RConn1 -- Cabinet2_4/LConn1
  5m25/RConn1 -- User14/LConn1
  5m23/RConn1 -- User12/LConn1
  10m26/RConn1 -- User16/LConn1
  10m22/RConn1 -- User11/LConn1
  Cable2_10m1/RConn2 -- Cabinet2_4/LConn2
  10m27/RConn1 -- User15/LConn1
  Cable2_10m1/RConn3 -- Cabinet2_4/LConn3
  Cable1_25m1/RConn1 -- Cabinet2_3/LConn1
  10m24/RConn1 -- User13/LConn1
  Cable1_25m1/RConn3 -- Cabinet2_3/LConn3
  Cable1_25m1/RConn2 -- Cabinet2_3/LConn2
  10m21/RConn1 -- User10/LConn1
  10+15m21/LConn1 -- User10/RConn1
  10+10m22/LConn1 -- User11/RConn1
  10+5m3/LConn1 -- User12/RConn1
  10+15m24/LConn1 -- User13/RConn1
  10+10m22/RConn1 -- 10+15m21/RConn1 -- 10+5m3/RConn1 -- 5+15m25/RConn1 -- 10+15m24/RConn1 -- Cabinet2_3/RConn4
  10+10m21/LConn1 -- User15/RConn1
  Cabinet2_4/RConn4 -- 10+5m23/RConn1 -- 10+10m21/RConn1
  10+5m7/LConn1 -- User9/RConn1
  User7/RConn1 -- 10+7m2/LConn1
  10+5m5/LConn1 -- User6/RConn1
  10+5m2/LConn1 -- User5/RConn1
  5+5m1/LConn1 -- User4/RConn1
  10+5m1/LConn1 -- User2/RConn1
  10+15m3/LConn1 -- User1/RConn1
  10+5m7/RConn1 -- 10+10m2/RConn1 -- 10+7m2/RConn1 -- 10+5m5/RConn1 -- Cabinet2_2/RConn4
  10+5m1/RConn1 -- 10+15m3/RConn1 -- 10+10m1/RConn1 -- 10+5m2/RConn1 -- 5+5m1/RConn1 -- Cabinet2_1/RConn4
  Cabinet2_1/LConn4 -- 30m2/RConn1
  Cabinet1_1/RConn4 -- 20m3/LConn1 -- 30m2/LConn1
  Cabinet1_1/LConn4 -- 3m2/RConn1
  3m5/RConn1 -- Cabinet1_2/LConn4
  Ground1/LConn1 -- Three-Phase Transformer (Two Windings)2/RConn4 -- 3m5/LConn1
  Cable1_15m3/RConn1 -- Three-Phase Transformer (Two Windings)/LConn1
  Cable1_15m3/RConn3 -- Three-Phase Transformer (Two Windings)/LConn3
  Three-Phase Transformer (Two Windings)/LConn2 -- Cable1_15m3/RConn2
  Cable1_15m4/RConn1 -- Three-Phase Transformer (Two Windings)2/LConn1
  Cable1_15m4/RConn2 -- Three-Phase Transformer (Two Windings)2/LConn2
  Cable1_15m4/RConn3 -- Three-Phase Transformer (Two Windings)2/LConn3
  Cable1_15m3/LConn1 -- Cable1_15m4/LConn1 -- Three-Phase Source/RConn1
  Cable1_15m3/LConn2 -- Cable1_15m4/LConn2 -- Three-Phase Source/RConn2
  Cable1_15m3/LConn3 -- Cable1_15m4/LConn3 -- Three-Phase Source/RConn3
  Three-Phase Transformer (Two Windings)/RConn1 -- Cable1_3m2/LConn1
  Three-Phase Transformer (Two Windings)/RConn2 -- Cable1_3m2/LConn2
  Three-Phase Transformer (Two Windings)/RConn3 -- Cable1_3m2/LConn3
  Cabinet1_1/LConn1 -- Cable1_3m2/RConn1
  Cabinet1_1/LConn2 -- Cable1_3m2/RConn2
  Cabinet1_1/LConn3 -- Cable1_3m2/RConn3
  Cable2_2m2/LConn2 -- Three-Phase Transformer (Two Windings)2/RConn2
  Three-Phase Transformer (Two Windings)2/RConn1 -- Cable2_2m2/LConn1
  Three-Phase Transformer (Two Windings)2/RConn3 -- Cable2_2m2/LConn3
  Cable2_2m2/RConn1 -- Cabinet1_2/LConn1
  Cable2_2m2/RConn2 -- Cabinet1_2/LConn2
  Cable2_2m2/RConn3 -- Cabinet1_2/LConn3
  Cable1_30m2/LConn2 -- Cable2_20m/LConn2 -- Cabinet1_1/RConn2
  Cabinet1_1/RConn3 -- Cable2_20m/LConn3 -- Cable1_30m2/LConn3
  Cabinet1_1/RConn1 -- Cable2_20m/LConn1 -- Cable1_30m2/LConn1
  Cable1_10m3/RConn1 -- 5m/LConn1
  10m1/LConn1 -- Cable1_10m3/RConn2
  Cable1_5m1/RConn3 -- 5m2/LConn1
  Cable1_5m1/RConn2 -- 10m2/LConn1
  Cable1_5m2/RConn1 -- 10m7/LConn1
  Cable1_15m1/RConn1 -- 10m21/LConn1
  Cabinet2_3/RConn1 -- Cable1_10m5/LConn1 -- Cable1_15m1/LConn1
  Cabinet2_3/RConn2 -- Cable1_10m5/LConn2 -- Cable1_15m1/LConn2
  Cabinet2_3/RConn3 -- Cable1_10m5/LConn3 -- Cable1_15m1/LConn3
  Cable1_10m5/RConn2 -- 10m22/LConn1
  Cable1_10m5/RConn3 -- 5m23/LConn1
  Cable1_15m5/LConn1 -- Cable1_5m7/LConn1 -- Cable1_10m6/LConn1 -- Cabinet2_4/RConn1
  Cable1_15m5/LConn2 -- Cable1_5m7/LConn2 -- Cable1_10m6/LConn2 -- Cabinet2_4/RConn2
  Cable1_15m5/LConn3 -- Cable1_5m7/LConn3 -- Cable1_10m6/LConn3 -- Cabinet2_4/RConn3
  Cable1_15m5/RConn1 -- 10m24/LConn1
  Cable1_15m5/RConn3 -- 5m25/LConn1
  Cable1_10m6/RConn2 -- 10m27/LConn1
  Cable1_5m7/RConn1 -- 10m26/LConn1
  Cable1_30m2/RConn1 -- Cabinet2_1/LConn1
  25m21/RConn1 -- Cabinet2_3/LConn4
  20m1/RConn1 -- Cabinet2_4/LConn4

== system Lv_topo4/Cabinet1_1 ==
  Three-Phase V-I Measurement : spsThreePhaseVIMeasurementLib/Three-Phase V-I Measurement  VoltageMeasurement=phase-to-ground  SetLabelV=on  LabelV=V_Cabinet1_1  Vpu=off  VpuLL=off  CurrentMeasurement=yes  SetLabelI=on  LabelI=I_Cabinet1_1  Ipu=off  Pbase=100e6  Vbase=500e3  OutputType=Complex  PhasorSimulation=off  PSBequivalent=0
  A : PMIOPort  Side=Left
  B : PMIOPort  Port=2  Side=Left
  C : PMIOPort  Port=3  Side=Left
  N : PMIOPort  Port=4  Side=Left
  A1 : PMIOPort  Port=5  Side=Right
  B1 : PMIOPort  Port=6  Side=Right
  C1 : PMIOPort  Port=7  Side=Right
  N1 : PMIOPort  Port=8  Side=Right
  connections:
  Three-Phase V-I Measurement/RConn1 -- A1/RConn1
  Three-Phase V-I Measurement/RConn2 -- B1/RConn1
  Three-Phase V-I Measurement/RConn3 -- C1/RConn1
  Three-Phase V-I Measurement/LConn1 -- A/RConn1
  B/RConn1 -- Three-Phase V-I Measurement/LConn2
  C/RConn1 -- Three-Phase V-I Measurement/LConn3
  N/RConn1 -- N1/RConn1

== system Lv_topo4/Cabinet1_2 ==
  Three-Phase V-I Measurement : spsThreePhaseVIMeasurementLib/Three-Phase V-I Measurement  VoltageMeasurement=phase-to-ground  SetLabelV=on  LabelV=V_Cabinet2_1  Vpu=off  VpuLL=off  CurrentMeasurement=yes  SetLabelI=on  LabelI=I_Cabinet2_1  Ipu=off  Pbase=100e6  Vbase=500e3  OutputType=Complex  PhasorSimulation=off  PSBequivalent=0
  A : PMIOPort  Side=Left
  B : PMIOPort  Port=2  Side=Left
  C : PMIOPort  Port=3  Side=Left
  N : PMIOPort  Port=4  Side=Left
  A1 : PMIOPort  Port=5  Side=Right
  B1 : PMIOPort  Port=6  Side=Right
  C1 : PMIOPort  Port=7  Side=Right
  N1 : PMIOPort  Port=8  Side=Right
  connections:
  Three-Phase V-I Measurement/RConn1 -- A1/RConn1
  Three-Phase V-I Measurement/RConn2 -- B1/RConn1
  Three-Phase V-I Measurement/RConn3 -- C1/RConn1
  Three-Phase V-I Measurement/LConn1 -- A/RConn1
  B/RConn1 -- Three-Phase V-I Measurement/LConn2
  C/RConn1 -- Three-Phase V-I Measurement/LConn3
  N/RConn1 -- N1/RConn1

== system Lv_topo4/Cabinet2_1 ==
  A : PMIOPort  Side=Left
  B : PMIOPort  Port=2  Side=Left
  C : PMIOPort  Port=3  Side=Left
  N : PMIOPort  Port=4  Side=Left
  Ao : PMIOPort  Port=5  Side=Right
  Bo : PMIOPort  Port=6  Side=Right
  Co : PMIOPort  Port=7  Side=Right
  No : PMIOPort  Port=8  Side=Right
  connections:
  A/RConn1 -- Ao/RConn1
  B/RConn1 -- Bo/RConn1
  C/RConn1 -- Co/RConn1
  N/RConn1 -- No/RConn1

== system Lv_topo4/Cabinet2_2 ==
  A : PMIOPort  Side=Left
  B : PMIOPort  Port=2  Side=Left
  C : PMIOPort  Port=3  Side=Left
  N : PMIOPort  Port=4  Side=Left
  Ao : PMIOPort  Port=5  Side=Right
  Bo : PMIOPort  Port=6  Side=Right
  Co : PMIOPort  Port=7  Side=Right
  No : PMIOPort  Port=8  Side=Right
  connections:
  A/RConn1 -- Ao/RConn1
  B/RConn1 -- Bo/RConn1
  C/RConn1 -- Co/RConn1
  N/RConn1 -- No/RConn1

== system Lv_topo4/Cabinet2_3 ==
  A : PMIOPort  Side=Left
  B : PMIOPort  Port=2  Side=Left
  C : PMIOPort  Port=3  Side=Left
  N : PMIOPort  Port=4  Side=Left
  Ao : PMIOPort  Port=5  Side=Right
  Bo : PMIOPort  Port=6  Side=Right
  Co : PMIOPort  Port=7  Side=Right
  No : PMIOPort  Port=8  Side=Right
  connections:
  A/RConn1 -- Ao/RConn1
  B/RConn1 -- Bo/RConn1
  C/RConn1 -- Co/RConn1
  N/RConn1 -- No/RConn1

== system Lv_topo4/Cabinet2_4 ==
  A : PMIOPort  Side=Left
  B : PMIOPort  Port=2  Side=Left
  C : PMIOPort  Port=3  Side=Left
  N : PMIOPort  Port=4  Side=Left
  Ao : PMIOPort  Port=5  Side=Right
  Bo : PMIOPort  Port=6  Side=Right
  Co : PMIOPort  Port=7  Side=Right
  No : PMIOPort  Port=8  Side=Right
  connections:
  A/RConn1 -- Ao/RConn1
  B/RConn1 -- Bo/RConn1
  C/RConn1 -- Co/RConn1
  N/RConn1 -- No/RConn1

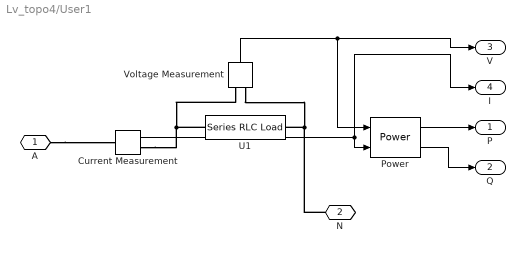
== system Lv_topo4/User1 ==
  Current Measurement : spsCurrentMeasurementLib/Current Measurement  PhasorSimulation=off  OutputType=Complex  PSBequivalent=0
  Power : spsPowerLib/Power  Freq=50  Vinit=[1, 0]  Iinit=[1, 0]  Ts=0
  U1 : spsSeriesRLCLoadLib/Series RLC Load  LConnTagsString=a  RConnTagsString=__new0  NominalVoltage=220  NominalFrequency=50  ActivePower=1171.8  InductivePower=682  CapacitivePower=0  Setx0=off  InitialVoltage=0  SetiL0=off  InitialCurrent=0  Measurements=None  LoadType=constant PQ
  Voltage Measurement : spsVoltageMeasurementLib/Voltage Measurement  PhasorSimulation=off  OutputType=Complex  PSBequivalent=0
  A : PMIOPort  Side=Left
  N : PMIOPort  Port=2  Side=Right
  P : Outport
  Q : Outport  Port=2
  V : Outport  Port=3
  I : Outport  Port=4
  wires:
  Power/1 -> P/1
  Power/2 -> Q/1
  Voltage Measurement/1 -> V/1, Power/1
  Current Measurement/1 -> Power/2, I/1
  connections:
  Voltage Measurement/LConn2 -- U1/RConn1 -- N/RConn1
  Voltage Measurement/LConn1 -- U1/LConn1 -- Current Measurement/RConn1
  A/RConn1 -- Current Measurement/LConn1

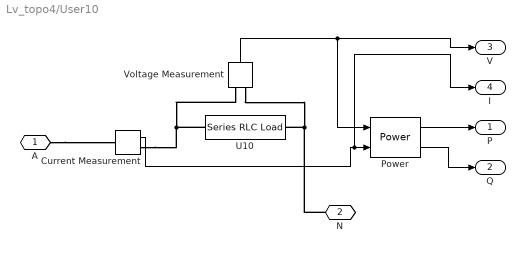
== system Lv_topo4/User10 ==
  Current Measurement : spsCurrentMeasurementLib/Current Measurement  PhasorSimulation=off  OutputType=Complex  PSBequivalent=0
  Power : spsPowerLib/Power  Freq=50  Vinit=[1, 0]  Iinit=[1, 0]  Ts=0
  U10 : spsSeriesRLCLoadLib/Series RLC Load  LConnTagsString=a  RConnTagsString=__new0  NominalVoltage=220  NominalFrequency=50  ActivePower=1600  InductivePower=880  CapacitivePower=0  Setx0=off  InitialVoltage=0  SetiL0=off  InitialCurrent=0  Measurements=None  LoadType=constant PQ
  Voltage Measurement : spsVoltageMeasurementLib/Voltage Measurement  PhasorSimulation=off  OutputType=Complex  PSBequivalent=0
  A : PMIOPort  Side=Left
  N : PMIOPort  Port=2  Side=Right
  P : Outport
  Q : Outport  Port=2
  V : Outport  Port=3
  I : Outport  Port=4
  wires:
  Power/1 -> P/1
  Power/2 -> Q/1
  Voltage Measurement/1 -> V/1, Power/1
  Current Measurement/1 -> I/1, Power/2
  connections:
  Voltage Measurement/LConn2 -- U10/RConn1 -- N/RConn1
  Voltage Measurement/LConn1 -- U10/LConn1 -- Current Measurement/RConn1
  A/RConn1 -- Current Measurement/LConn1

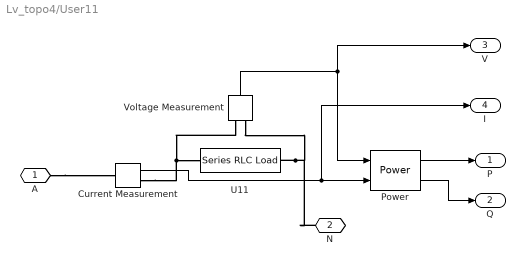
== system Lv_topo4/User11 ==
  Current Measurement : spsCurrentMeasurementLib/Current Measurement  PhasorSimulation=off  OutputType=Complex  PSBequivalent=0
  Power : spsPowerLib/Power  Freq=50  Vinit=[1, 0]  Iinit=[1, 0]  Ts=0
  U11 : spsSeriesRLCLoadLib/Series RLC Load  LConnTagsString=a  RConnTagsString=__new0  NominalVoltage=220  NominalFrequency=50  ActivePower=1125  InductivePower=585  CapacitivePower=0  Setx0=off  InitialVoltage=0  SetiL0=off  InitialCurrent=0  Measurements=None  LoadType=constant PQ
  Voltage Measurement : spsVoltageMeasurementLib/Voltage Measurement  PhasorSimulation=off  OutputType=Complex  PSBequivalent=0
  A : PMIOPort  Side=Left
  N : PMIOPort  Port=2  Side=Right
  P : Outport
  Q : Outport  Port=2
  V : Outport  Port=3
  I : Outport  Port=4
  wires:
  Power/1 -> P/1
  Power/2 -> Q/1
  Voltage Measurement/1 -> V/1, Power/1
  Current Measurement/1 -> I/1, Power/2
  connections:
  U11/RConn1 -- Voltage Measurement/LConn2 -- N/RConn1
  Current Measurement/RConn1 -- Voltage Measurement/LConn1 -- U11/LConn1
  A/RConn1 -- Current Measurement/LConn1

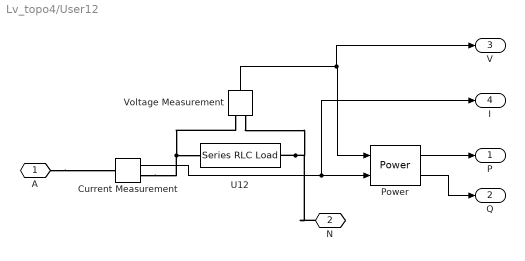
== system Lv_topo4/User12 ==
  Current Measurement : spsCurrentMeasurementLib/Current Measurement  PhasorSimulation=off  OutputType=Complex  PSBequivalent=0
  Power : spsPowerLib/Power  Freq=50  Vinit=[1, 0]  Iinit=[1, 0]  Ts=0
  U12 : spsSeriesRLCLoadLib/Series RLC Load  LConnTagsString=a  RConnTagsString=__new0  NominalVoltage=220  NominalFrequency=50  ActivePower=1160  InductivePower=568  CapacitivePower=0  Setx0=off  InitialVoltage=0  SetiL0=off  InitialCurrent=0  Measurements=None  LoadType=constant PQ
  Voltage Measurement : spsVoltageMeasurementLib/Voltage Measurement  PhasorSimulation=off  OutputType=Complex  PSBequivalent=0
  A : PMIOPort  Side=Left
  N : PMIOPort  Port=2  Side=Right
  P : Outport
  Q : Outport  Port=2
  V : Outport  Port=3
  I : Outport  Port=4
  wires:
  Power/1 -> P/1
  Power/2 -> Q/1
  Current Measurement/1 -> I/1, Power/2
  Voltage Measurement/1 -> V/1, Power/1
  connections:
  U12/RConn1 -- Voltage Measurement/LConn2 -- N/RConn1
  Current Measurement/RConn1 -- Voltage Measurement/LConn1 -- U12/LConn1
  A/RConn1 -- Current Measurement/LConn1

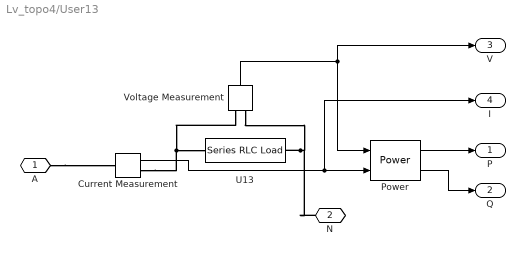
== system Lv_topo4/User13 ==
  Current Measurement : spsCurrentMeasurementLib/Current Measurement  PhasorSimulation=off  OutputType=Complex  PSBequivalent=0
  Power : spsPowerLib/Power  Freq=50  Vinit=[1, 0]  Iinit=[1, 0]  Ts=0
  U13 : spsSeriesRLCLoadLib/Series RLC Load  LConnTagsString=a  RConnTagsString=__new0  NominalVoltage=220  NominalFrequency=50  ActivePower=951.5  InductivePower=429  CapacitivePower=0  Setx0=off  InitialVoltage=0  SetiL0=off  InitialCurrent=0  Measurements=None  LoadType=constant PQ
  Voltage Measurement : spsVoltageMeasurementLib/Voltage Measurement  PhasorSimulation=off  OutputType=Complex  PSBequivalent=0
  A : PMIOPort  Side=Left
  N : PMIOPort  Port=2  Side=Right
  P : Outport
  Q : Outport  Port=2
  V : Outport  Port=3
  I : Outport  Port=4
  wires:
  Power/1 -> P/1
  Power/2 -> Q/1
  Voltage Measurement/1 -> V/1, Power/1
  Current Measurement/1 -> I/1, Power/2
  connections:
  U13/RConn1 -- Voltage Measurement/LConn2 -- N/RConn1
  Current Measurement/RConn1 -- Voltage Measurement/LConn1 -- U13/LConn1
  A/RConn1 -- Current Measurement/LConn1

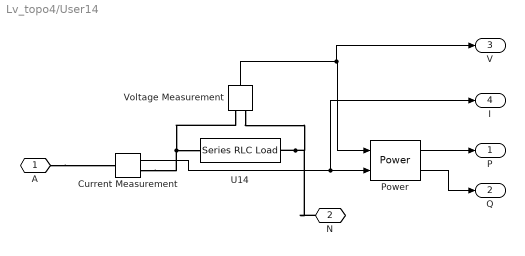
== system Lv_topo4/User14 ==
  Current Measurement : spsCurrentMeasurementLib/Current Measurement  PhasorSimulation=off  OutputType=Complex  PSBequivalent=0
  Power : spsPowerLib/Power  Freq=50  Vinit=[1, 0]  Iinit=[1, 0]  Ts=0
  U14 : spsSeriesRLCLoadLib/Series RLC Load  LConnTagsString=a  RConnTagsString=__new0  NominalVoltage=220  NominalFrequency=50  ActivePower=896.5  InductivePower=415.25  CapacitivePower=0  Setx0=off  InitialVoltage=0  SetiL0=off  InitialCurrent=0  Measurements=None  LoadType=constant PQ
  Voltage Measurement : spsVoltageMeasurementLib/Voltage Measurement  PhasorSimulation=off  OutputType=Complex  PSBequivalent=0
  A : PMIOPort  Side=Left
  N : PMIOPort  Port=2  Side=Right
  P : Outport
  Q : Outport  Port=2
  V : Outport  Port=3
  I : Outport  Port=4
  wires:
  Power/1 -> P/1
  Power/2 -> Q/1
  Current Measurement/1 -> I/1, Power/2
  Voltage Measurement/1 -> V/1, Power/1
  connections:
  U14/RConn1 -- Voltage Measurement/LConn2 -- N/RConn1
  Current Measurement/RConn1 -- Voltage Measurement/LConn1 -- U14/LConn1
  A/RConn1 -- Current Measurement/LConn1
